simulink model "DCCurrentEstimationslx"  (R2022b)
settings: Solver=ode1  StartTime=0.0  StopTime=0.2  FixedStep=ctrlConst.TsSwitch  MaxStep=1e-6  RelTol=1e-3  EnableMultiTasking=on
undefined symbols (not defined in the file or in its folder): DeadPrd_P, f32_P_Tonoff, f32_P_Tonoff2, Ts
libraries: simulink x5
settings Model: Creator=M00039784  LastModifiedBy=M00039784
settings SolverCC: AlgebraicLoopSolver=TrustRegion  InsertRTBMode=Never (minimum delay)
settings DataIOCC: LimitDataPoints=on  SaveFormat=Array  SaveOutput=off  SaveTime=off
settings OptimizationCC: DefaultParameterBehavior=Inlined  UseDivisionForNetSlopeComputation=on  UseFloatMulNetSlope=on  DefaultUnderspecifiedDataType=single  InlineInvariantSignals=on  PassReuseOutputArgsAs=Individual arguments  ExpressionDepthLimit=2147483647  ZeroExternalMemoryAtStartup=off  ZeroInternalMemoryAtStartup=off  NoFixptDivByZeroProtection=on  EfficientFloat2IntCast=on  LifeSpan=1  EfficientTunableParamExpr=on
settings DebuggingCC: ReadBeforeWriteMsg=DisableAll  WriteAfterWriteMsg=DisableAll  WriteAfterReadMsg=DisableAll  AlgebraicLoopMsg=none  MultiTaskDSMMsg=none  SingleTaskRateTransMsg=error  IntegerOverflowMsg=none  ParameterPrecisionLossMsg=none  FcnCallInpInsideContextMsg=warning  BusObjectLabelMismatch=none  AssertControl=DisableAll  AllowSymbolicDim=off  StateNameClashWarn=warning  SFUnexpectedBacktrackingDiag=warning  SFNoUnconditionalDefaultTransitionDiag=warning  SFExecutionAtInitializationDiag=none  SFMachineParentedDataDiag=warning  IntegerSaturationMsg=none  UnitsInconsistencyMsg=none  ArithmeticOperatorsInVariantConditions=warning
settings HardwareCC: ProdBitPerPointer=32  ProdBitPerSizeT=32  ProdBitPerPtrDiffT=32  ProdLargestAtomicFloat=None  ProdWordSize=32  ProdHWDeviceType=Infineon->TriCore
settings ModelReferenceCC: UpdateModelReferenceTargets=IfOutOfDate  EnableRefExpFcnMdlSchedulingChecks=on  ModelReferenceNumInstancesAllowed=Single  PropagateSignalLabelsOutOfModel=off
settings SFSimCC: SFSimEcho=off  SimUseLocalCustomCode=off  MATLABDynamicMemAlloc=off  CustomCodeUndefinedFunction=UseInterfaceOnly
settings RTWCC: Description=Embedded Coder  SystemTargetFile=ert.tlc  GenCodeOnly=on  GenerateMakefile=off  TemplateMakefile=ec_target.tmf  RTWVerbose=off  RTWUseLocalCustomCode=off  PortableWordSizes=on  CodeExecutionProfiling=on  CodeProfilingSaveOptions=AllData  CodeProfilingInstrumentation=detailed
settings CodeAppCC: ForceParamTrailComments=on  IgnoreCustomStorageClasses=off  IgnoreTestpoints=on  MaxIdLength=64  SimulinkDataObjDesc=on  MATLABFcnDesc=on  CustomSymbolStrGlobalVar=pmsmfoc_rt$N$M  CustomSymbolStrType=pmsmfoc_$N$M  CustomSymbolStrFcn=$N$M$F  CustomSymbolStrFcnArg=$I$N$M  CustomSymbolStrMacro=$N$M  InsertBlockDesc=on  StateflowObjectComments=on  MATLABSourceComments=on  InternalIdentifier=Classic
settings ERTTargetCC: UtilityFuncGeneration=Shared location  MultiwordLength=2048  CombineSignalStateStructs=on  SupportAbsoluteTime=off  SupportNonFinite=off  SupportComplex=off  SupportNonInlinedSFcns=on  RemoveResetFunc=off  ParenthesesLevel=Maximum  GenerateASAP2=on  InlinedParameterPlacement=NonHierarchical  ERTCustomFileTemplate=example_file_process.tlc  EnableDataOwnership=on  ConvertIfToSwitch=off  SuppressUnreachableDefaultCases=off  MemSecPackage=Simulink  MemSecDataConstants=MemConst  MemSecDataParameters=MemConstVolatile
settings ConfigComp: CovMetricSettings=dcmtrzow  CovHTMLOptions=-aTS=1 -bRG=1 -bTC=1 -hTR=0 -nFC=0 -scm=1 -bcm=1 -xEv=0  CovSaveCumulativeToWorkspaceVar=on  CovSaveSingleToWorkspaceVar=on  CovExternalEMLEnable=off  CovSFcnEnable=off
settings SimscapeCC: SimscapeNormalizeSystem=off

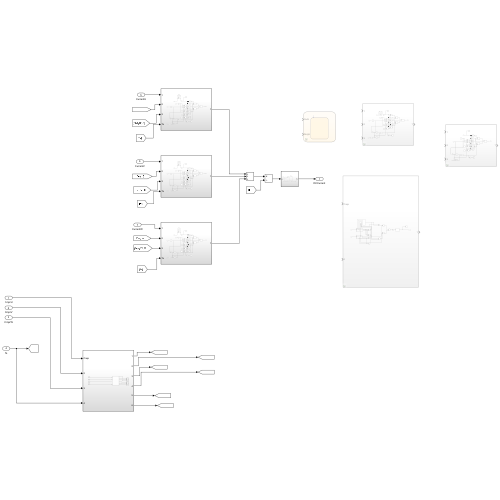
[thumbnail: Simulink's stored preview of the top-level diagram]
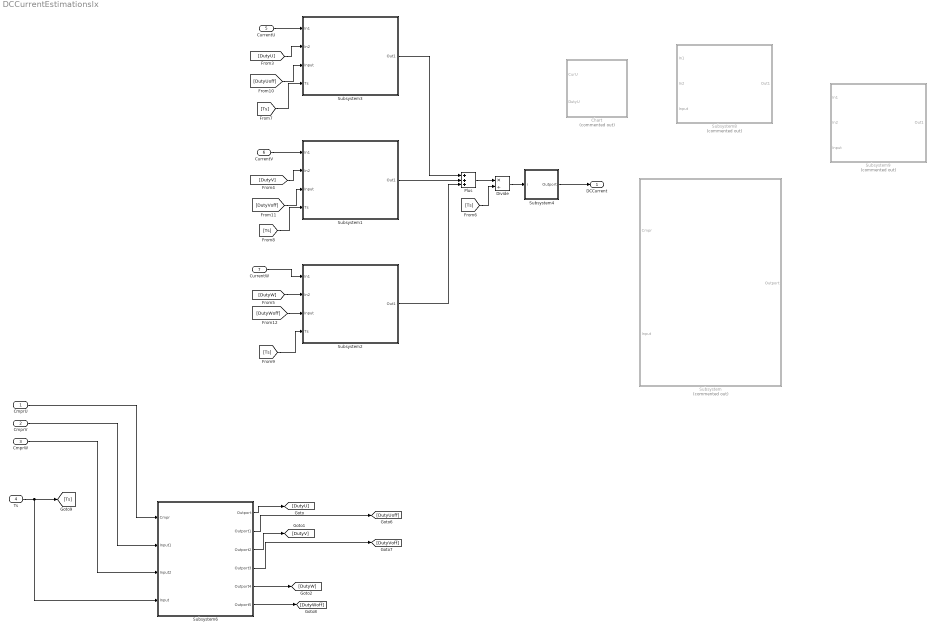
== system DCCurrentEstimationslx ==
  CmprU : Inport  OutDataTypeStr=single  PortDimensions=1  SampleTime=[0.0001,0]
  CmprV : Inport  Port=2  OutDataTypeStr=single
  CmprW : Inport  Port=3  OutDataTypeStr=single
  Ts : Inport  Port=4  OutDataTypeStr=single  PortDimensions=1  SampleTime=[0.0001,0]
  CurrentU : Inport  Port=5  OutDataTypeStr=single
  CurrentV : Inport  Port=6  OutDataTypeStr=single
  CurrentW : Inport  Port=7  OutDataTypeStr=single
  Chart : Stateflow chart  Commented=on  TreatAsAtomicUnit=on
  Divide : Product  Inputs=*/  OutDataTypeStr=single
  Plus : Sum  Inputs=+++
  Subsystem : Subsystem  Commented=on
  Subsystem1 : Subsystem
  Subsystem2 : Subsystem
  Subsystem3 : Subsystem
  Subsystem4 : Subsystem
  Subsystem6 : Subsystem
  Subsystem8 : Subsystem  Commented=on
  Subsystem9 : Subsystem  Commented=on
  DCCurrent : Outport  OutDataTypeStr=single  PortDimensions=1  SampleTime=[0.0001,0]
  wires:
  [DutyU] -> Subsystem3/2(In2)
  CurrentU/1 -> Subsystem3/1(In1)
  CurrentV/1 -> Subsystem1/1(In1)
  [DutyV] -> Subsystem1/2(In2)
  Subsystem1/1(Out1) -> Plus/2
  Plus/1 -> Divide/1
  CurrentW/1 -> Subsystem2/1(In1)
  [DutyW] -> Subsystem2/2(In2)
  Subsystem2/1(Out1) -> Plus/3
  Divide/1 -> Subsystem4/1(i)
  Subsystem4/1(Outport) -> DCCurrent/1
  Subsystem3/1(Out1) -> Plus/1
  [DutyUoff] -> Subsystem3/3(Input)
  [DutyVoff] -> Subsystem1/3(Input)
  [DutyWoff] -> Subsystem2/3(Input)
  Ts/1 -> Subsystem6/4(Input), [Ts]
  [Ts] -> Divide/2
  [Ts] -> Subsystem2/4(Ts)
  [Ts] -> Subsystem3/4(Ts)
  [Ts] -> Subsystem1/4(Ts)
  CmprU/1 -> Subsystem6/1(Cmpr)
  CmprV/1 -> Subsystem6/2(Input1)
  CmprW/1 -> Subsystem6/3(Input2)
  Subsystem6/5(Outport4) -> [DutyW]
  Subsystem6/3(Outport2) -> [DutyV]
  Subsystem6/1(Outport) -> [DutyU]
  Subsystem6/2(Outport1) -> [DutyUoff]
  Subsystem6/4(Outport3) -> [DutyVoff]
  Subsystem6/6(Outport5) -> [DutyWoff]

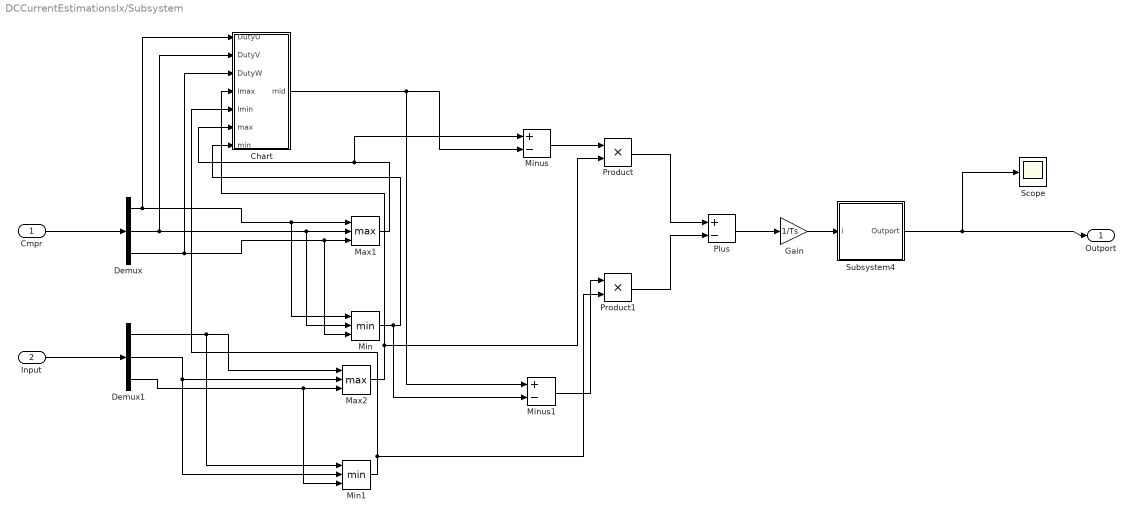
== system DCCurrentEstimationslx/Subsystem ==
  Cmpr : Inport
  Input : Inport  Port=2
  Chart : Stateflow chart  TreatAsAtomicUnit=on
  Demux : Demux  Outputs=3
  Demux1 : Demux  Outputs=3
  Gain : Gain  Gain=1/Ts
  Max1 : MinMax  Function=max  Inputs=3
  Max2 : MinMax  Function=max  Inputs=3
  Min : MinMax  Inputs=3
  Min1 : MinMax  Inputs=3
  Minus : Sum  Inputs=+-
  Minus1 : Sum  Inputs=+-
  Plus : Sum  Inputs=+-
  Product : Product
  Product1 : Product
  Scope : Scope
  Subsystem4 : Subsystem
  Outport : Outport
  wires:
  Subsystem4/1(Outport) -> Outport/1, Scope/1
  Gain/1 -> Subsystem4/1(i)
  Plus/1 -> Gain/1
  Product1/1 -> Plus/2
  Product/1 -> Plus/1
  Minus1/1 -> Product1/1
  Minus/1 -> Product/1
  Chart/1(mid) -> Minus/2, Minus1/1
  Min1/1 -> Chart/5(Imin), Product1/2
  Max2/1 -> Chart/4(Imax), Product/2
  Demux1/1 -> Max2/1, Min1/1
  Demux1/2 -> Max2/2, Min1/2
  Demux1/3 -> Min1/3, Max2/3
  Max1/1 -> Chart/6(max), Minus/1
  Min/1 -> Chart/7(min), Minus1/2
  Demux/1 -> Max1/1, Min/1, Chart/1(DutyU)
  Demux/2 -> Min/2, Max1/2, Chart/2(DutyV)
  Demux/3 -> Max1/3, Min/3, Chart/3(DutyW)
  Input/1 -> Demux1/1
  Cmpr/1 -> Demux/1

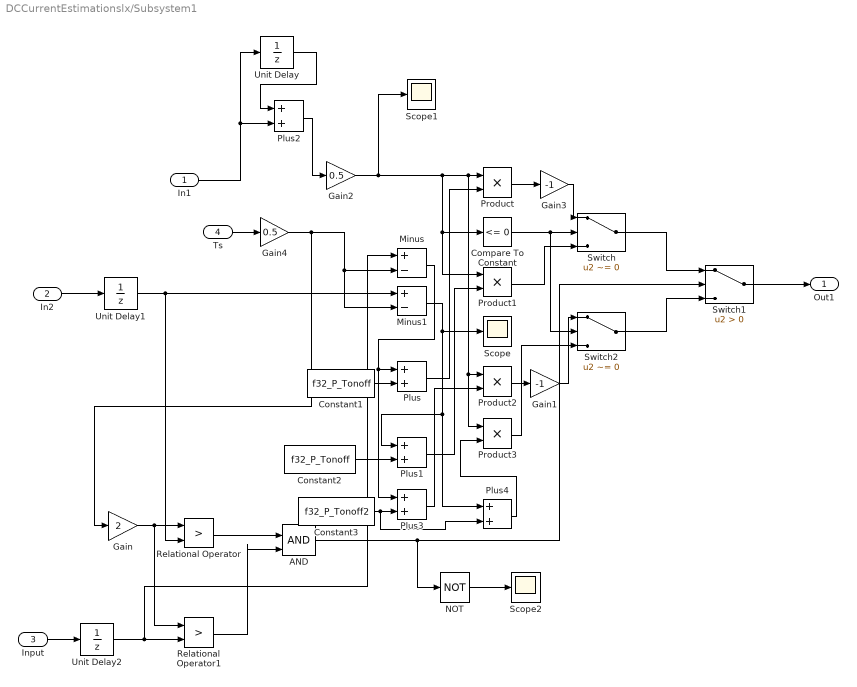
== system DCCurrentEstimationslx/Subsystem1 ==
  In1 : Inport
  In2 : Inport  Port=2
  Input : Inport  Port=3
  Ts : Inport  Port=4
  AND : Logic  IconShape=distinctive  AllPortsSameDT=off  OutDataTypeStr=boolean
  Compare To Constant : simulink/Logic and Bit Operations/Compare To Constant  relop=<=  const=0  OutDataTypeStr=boolean
  Constant1 : Constant  Value=f32_P_Tonoff  OutDataTypeStr=single
  Constant2 : Constant  Value=f32_P_Tonoff  OutDataTypeStr=single
  Constant3 : Constant  Value=f32_P_Tonoff2  OutDataTypeStr=single
  Gain : Gain  Gain=2
  Gain1 : Gain  Gain=-1
  Gain2 : Gain  Gain=0.5
  Gain3 : Gain  Gain=-1
  Gain4 : Gain  Gain=0.5
  Minus : Sum  Inputs=+-
  Minus1 : Sum  Inputs=+-
  NOT : Logic  Operator=NOT  IconShape=distinctive  AllPortsSameDT=off  OutDataTypeStr=boolean
  Plus{,1..4} (5 alike) : Sum
  Product{,1..3} (4 alike) : Product
  Relational Operator : RelationalOperator  Operator=>  OutDataTypeStr=boolean  RndMeth=Simplest  InputSameDT=off
  Relational Operator1 : RelationalOperator  Operator=>  OutDataTypeStr=boolean  RndMeth=Simplest  InputSameDT=off
  Scope : Scope
  Scope1 : Scope
  Scope2 : Scope
  Switch : Switch  Criteria=u2 ~= 0  SaturateOnIntegerOverflow=off  InputSameDT=off
  Switch1 : Switch  Criteria=u2 > Threshold  SaturateOnIntegerOverflow=off  InputSameDT=off
  Switch2 : Switch  Criteria=u2 ~= 0  SaturateOnIntegerOverflow=off  InputSameDT=off
  Unit Delay : UnitDelay  SampleTime=-1  HasFrameUpgradeWarning=on
  Unit Delay1 : UnitDelay  SampleTime=-1  HasFrameUpgradeWarning=on
  Unit Delay2 : UnitDelay  SampleTime=-1  HasFrameUpgradeWarning=on
  Out1 : Outport
  wires:
  Ts/1 -> Gain4/1
  Plus4/1 -> Product3/2
  Plus3/1 -> Product2/2
  Constant3/1 -> Plus3/2, Plus4/2
  Switch2/1 -> Switch1/3
  Plus/1 -> Product/2
  Gain3/1 -> Switch/1
  In1/1 -> Plus2/2, Unit Delay/1
  Unit Delay2/1 -> Relational Operator1/2, Minus/1
  Unit Delay1/1 -> Relational Operator/2, Minus1/1
  Plus2/1 -> Gain2/1
  Unit Delay/1 -> Plus2/1
  NOT/1 -> Scope2/1
  Product3/1 -> Switch2/3
  Gain1/1 -> Switch2/1
  Product2/1 -> Gain1/1
  Switch1/1 -> Out1/1
  Relational Operator1/1 -> AND/2
  Input/1 -> Unit Delay2/1
  Relational Operator/1 -> AND/1
  AND/1 -> Switch1/2, NOT/1
  Gain/1 -> Relational Operator/1, Relational Operator1/1
  Plus1/1 -> Product1/2
  Minus1/1 -> Plus1/1, Plus4/1, Scope/1
  Constant2/1 -> Plus1/2
  Constant1/1 -> Plus/2
  Product1/1 -> Switch/3
  Minus/1 -> Plus3/1, Plus/1
  Compare To Constant/1 -> Switch/2, Switch2/2
  Gain2/1 -> Product/1, Product3/1, Product2/1, Compare To Constant/1, Product1/1, Scope1/1
  Product/1 -> Gain3/1
  Gain4/1 -> Minus1/2, Minus/2, Gain/1
  Switch/1 -> Switch1/1
  In2/1 -> Unit Delay1/1

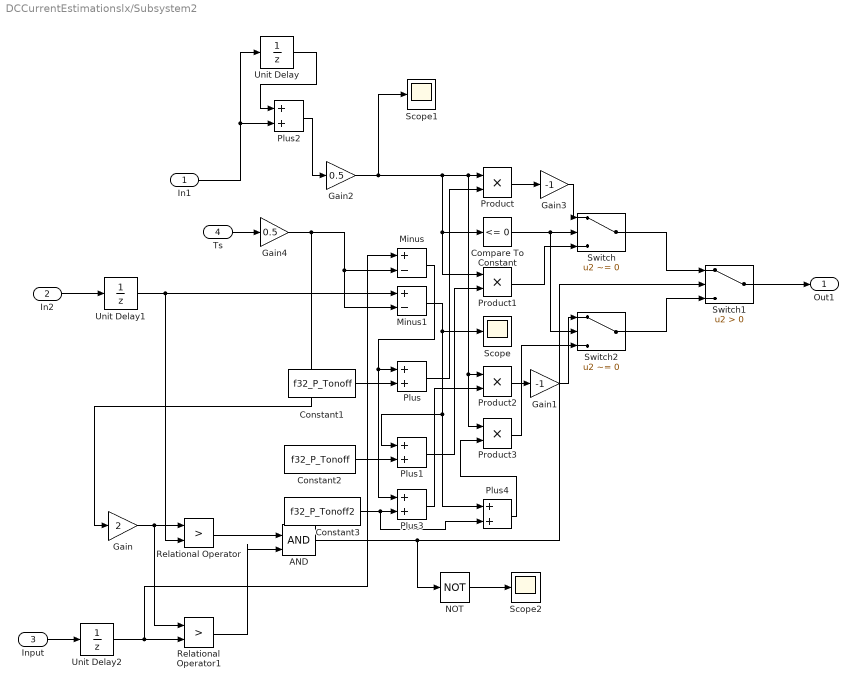
== system DCCurrentEstimationslx/Subsystem2 ==
  In1 : Inport
  In2 : Inport  Port=2
  Input : Inport  Port=3
  Ts : Inport  Port=4
  AND : Logic  IconShape=distinctive  AllPortsSameDT=off  OutDataTypeStr=boolean
  Compare To Constant : simulink/Logic and Bit Operations/Compare To Constant  relop=<=  const=0  OutDataTypeStr=boolean
  Constant1 : Constant  Value=f32_P_Tonoff  OutDataTypeStr=single
  Constant2 : Constant  Value=f32_P_Tonoff  OutDataTypeStr=single
  Constant3 : Constant  Value=f32_P_Tonoff2  OutDataTypeStr=single
  Gain : Gain  Gain=2
  Gain1 : Gain  Gain=-1
  Gain2 : Gain  Gain=0.5
  Gain3 : Gain  Gain=-1
  Gain4 : Gain  Gain=0.5
  Minus : Sum  Inputs=+-
  Minus1 : Sum  Inputs=+-
  NOT : Logic  Operator=NOT  IconShape=distinctive  AllPortsSameDT=off  OutDataTypeStr=boolean
  Plus{,1..4} (5 alike) : Sum
  Product{,1..3} (4 alike) : Product
  Relational Operator : RelationalOperator  Operator=>  OutDataTypeStr=boolean  RndMeth=Simplest  InputSameDT=off
  Relational Operator1 : RelationalOperator  Operator=>  OutDataTypeStr=boolean  RndMeth=Simplest  InputSameDT=off
  Scope : Scope
  Scope1 : Scope
  Scope2 : Scope
  Switch : Switch  Criteria=u2 ~= 0  SaturateOnIntegerOverflow=off  InputSameDT=off
  Switch1 : Switch  Criteria=u2 > Threshold  SaturateOnIntegerOverflow=off  InputSameDT=off
  Switch2 : Switch  Criteria=u2 ~= 0  SaturateOnIntegerOverflow=off  InputSameDT=off
  Unit Delay : UnitDelay  SampleTime=-1  HasFrameUpgradeWarning=on
  Unit Delay1 : UnitDelay  SampleTime=-1  HasFrameUpgradeWarning=on
  Unit Delay2 : UnitDelay  SampleTime=-1  HasFrameUpgradeWarning=on
  Out1 : Outport
  wires:
  Ts/1 -> Gain4/1
  Plus4/1 -> Product3/2
  Plus3/1 -> Product2/2
  Constant3/1 -> Plus3/2, Plus4/2
  Switch2/1 -> Switch1/3
  Plus/1 -> Product/2
  Gain3/1 -> Switch/1
  In1/1 -> Plus2/2, Unit Delay/1
  Unit Delay2/1 -> Relational Operator1/2, Minus/1
  Unit Delay1/1 -> Relational Operator/2, Minus1/1
  Plus2/1 -> Gain2/1
  Unit Delay/1 -> Plus2/1
  NOT/1 -> Scope2/1
  Product3/1 -> Switch2/3
  Gain1/1 -> Switch2/1
  Product2/1 -> Gain1/1
  Switch1/1 -> Out1/1
  Relational Operator1/1 -> AND/2
  Input/1 -> Unit Delay2/1
  Relational Operator/1 -> AND/1
  AND/1 -> Switch1/2, NOT/1
  Gain/1 -> Relational Operator/1, Relational Operator1/1
  Plus1/1 -> Product1/2
  Minus1/1 -> Plus1/1, Plus4/1, Scope/1
  Constant2/1 -> Plus1/2
  Constant1/1 -> Plus/2
  Product1/1 -> Switch/3
  Minus/1 -> Plus3/1, Plus/1
  Compare To Constant/1 -> Switch/2, Switch2/2
  Gain2/1 -> Product/1, Product3/1, Product2/1, Compare To Constant/1, Product1/1, Scope1/1
  Product/1 -> Gain3/1
  Gain4/1 -> Minus1/2, Minus/2, Gain/1
  Switch/1 -> Switch1/1
  In2/1 -> Unit Delay1/1

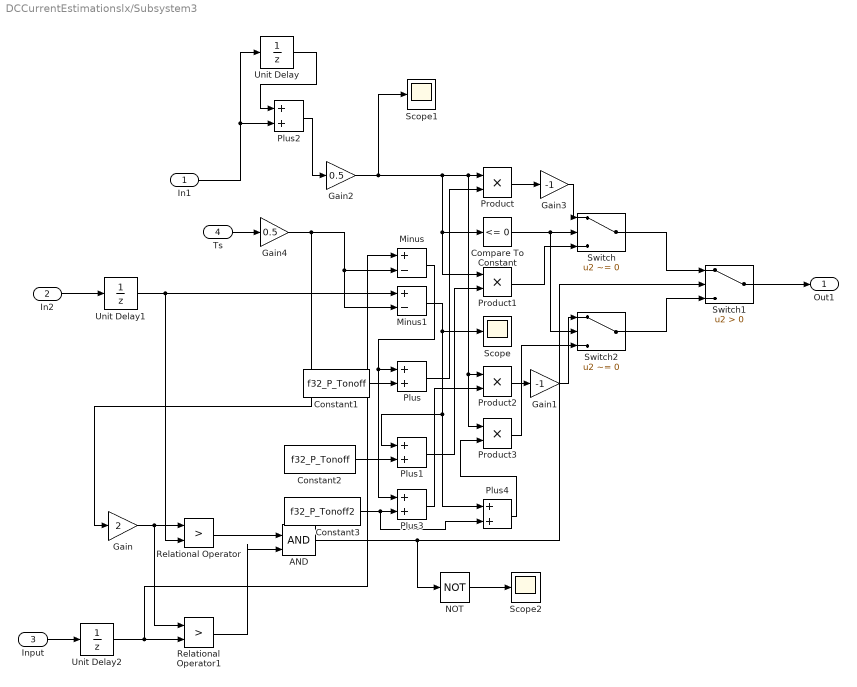
== system DCCurrentEstimationslx/Subsystem3 ==
  In1 : Inport
  In2 : Inport  Port=2
  Input : Inport  Port=3
  Ts : Inport  Port=4
  AND : Logic  IconShape=distinctive  AllPortsSameDT=off  OutDataTypeStr=boolean
  Compare To Constant : simulink/Logic and Bit Operations/Compare To Constant  relop=<=  const=0  OutDataTypeStr=boolean
  Constant1 : Constant  Value=f32_P_Tonoff  OutDataTypeStr=single
  Constant2 : Constant  Value=f32_P_Tonoff  OutDataTypeStr=single
  Constant3 : Constant  Value=f32_P_Tonoff2  OutDataTypeStr=single
  Gain : Gain  Gain=2
  Gain1 : Gain  Gain=-1
  Gain2 : Gain  Gain=0.5
  Gain3 : Gain  Gain=-1
  Gain4 : Gain  Gain=0.5
  Minus : Sum  Inputs=+-
  Minus1 : Sum  Inputs=+-
  NOT : Logic  Operator=NOT  IconShape=distinctive  AllPortsSameDT=off  OutDataTypeStr=boolean
  Plus{,1..4} (5 alike) : Sum
  Product{,1..3} (4 alike) : Product
  Relational Operator : RelationalOperator  Operator=>  OutDataTypeStr=boolean  RndMeth=Simplest  InputSameDT=off
  Relational Operator1 : RelationalOperator  Operator=>  OutDataTypeStr=boolean  RndMeth=Simplest  InputSameDT=off
  Scope : Scope
  Scope1 : Scope
  Scope2 : Scope
  Switch : Switch  Criteria=u2 ~= 0  SaturateOnIntegerOverflow=off  InputSameDT=off
  Switch1 : Switch  Criteria=u2 > Threshold  SaturateOnIntegerOverflow=off  InputSameDT=off
  Switch2 : Switch  Criteria=u2 ~= 0  SaturateOnIntegerOverflow=off  InputSameDT=off
  Unit Delay : UnitDelay  SampleTime=-1  HasFrameUpgradeWarning=on
  Unit Delay1 : UnitDelay  SampleTime=-1  HasFrameUpgradeWarning=on
  Unit Delay2 : UnitDelay  SampleTime=-1  HasFrameUpgradeWarning=on
  Out1 : Outport
  wires:
  Ts/1 -> Gain4/1
  Plus4/1 -> Product3/2
  Plus3/1 -> Product2/2
  Constant3/1 -> Plus3/2, Plus4/2
  Switch2/1 -> Switch1/3
  Plus/1 -> Product/2
  Gain3/1 -> Switch/1
  In1/1 -> Plus2/2, Unit Delay/1
  Unit Delay2/1 -> Relational Operator1/2, Minus/1
  Unit Delay1/1 -> Relational Operator/2, Minus1/1
  Plus2/1 -> Gain2/1
  Unit Delay/1 -> Plus2/1
  NOT/1 -> Scope2/1
  Product3/1 -> Switch2/3
  Gain1/1 -> Switch2/1
  Product2/1 -> Gain1/1
  Switch1/1 -> Out1/1
  Relational Operator1/1 -> AND/2
  Input/1 -> Unit Delay2/1
  Relational Operator/1 -> AND/1
  AND/1 -> Switch1/2, NOT/1
  Gain/1 -> Relational Operator/1, Relational Operator1/1
  Plus1/1 -> Product1/2
  Minus1/1 -> Plus1/1, Plus4/1, Scope/1
  Constant2/1 -> Plus1/2
  Constant1/1 -> Plus/2
  Product1/1 -> Switch/3
  Minus/1 -> Plus3/1, Plus/1
  Compare To Constant/1 -> Switch/2, Switch2/2
  Gain2/1 -> Product/1, Product3/1, Product2/1, Compare To Constant/1, Product1/1, Scope1/1
  Product/1 -> Gain3/1
  Gain4/1 -> Minus1/2, Minus/2, Gain/1
  Switch/1 -> Switch1/1
  In2/1 -> Unit Delay1/1

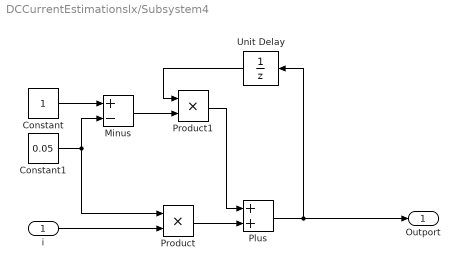
== system DCCurrentEstimationslx/Subsystem4 ==
  i : Inport
  Constant : Constant  OutDataTypeStr=single
  Constant1 : Constant  Value=0.05  OutDataTypeStr=single
  Minus : Sum  Inputs=+-
  Plus : Sum
  Product : Product
  Product1 : Product
  Unit Delay : UnitDelay  SampleTime=-1  HasFrameUpgradeWarning=on
  Outport : Outport
  wires:
  Unit Delay/1 -> Product1/1
  Plus/1 -> Outport/1, Unit Delay/1
  Product1/1 -> Plus/1
  Minus/1 -> Product1/2
  Product/1 -> Plus/2
  i/1 -> Product/2
  Constant1/1 -> Minus/2, Product/1
  Constant/1 -> Minus/1

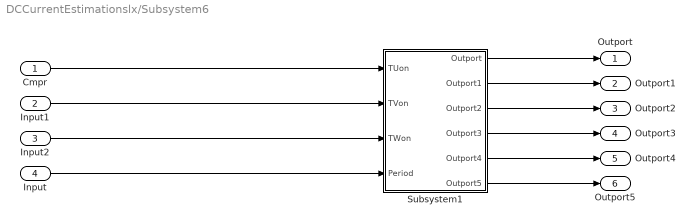
== system DCCurrentEstimationslx/Subsystem6 ==
  Cmpr : Inport
  Input1 : Inport  Port=2
  Input2 : Inport  Port=3
  Input : Inport  Port=4
  Subsystem1 : Subsystem
  Outport : Outport
  Outport1 : Outport  Port=2
  Outport2 : Outport  Port=3
  Outport3 : Outport  Port=4
  Outport4 : Outport  Port=5
  Outport5 : Outport  Port=6
  wires:
  Subsystem1/6(Outport5) -> Outport5/1
  Subsystem1/5(Outport4) -> Outport4/1
  Subsystem1/4(Outport3) -> Outport3/1
  Subsystem1/3(Outport2) -> Outport2/1
  Subsystem1/2(Outport1) -> Outport1/1
  Subsystem1/1(Outport) -> Outport/1
  Input/1 -> Subsystem1/4(Period)
  Input2/1 -> Subsystem1/3(TWon)
  Input1/1 -> Subsystem1/2(TVon)
  Cmpr/1 -> Subsystem1/1(TUon)

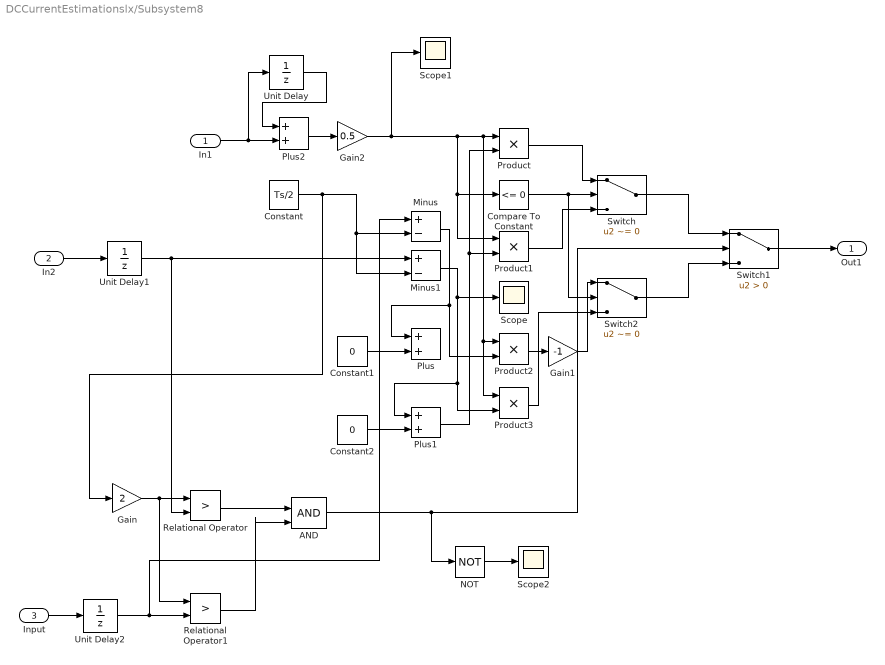
== system DCCurrentEstimationslx/Subsystem8 ==
  In1 : Inport
  In2 : Inport  Port=2
  Input : Inport  Port=3
  AND : Logic  IconShape=distinctive  AllPortsSameDT=off  OutDataTypeStr=boolean
  Compare To Constant : simulink/Logic and Bit Operations/Compare To Constant  relop=<=  const=0  OutDataTypeStr=boolean
  Constant : Constant  Value=Ts/2
  Constant1 : Constant  Value=0
  Constant2 : Constant  Value=0
  Gain : Gain  Gain=2
  Gain1 : Gain  Gain=-1
  Gain2 : Gain  Gain=0.5
  Minus : Sum  Inputs=+-
  Minus1 : Sum  Inputs=+-
  NOT : Logic  Operator=NOT  IconShape=distinctive  AllPortsSameDT=off  OutDataTypeStr=boolean
  Plus : Sum
  Plus1 : Sum
  Plus2 : Sum
  Product{,1..3} (4 alike) : Product
  Relational Operator : RelationalOperator  Operator=>  OutDataTypeStr=boolean  RndMeth=Simplest  InputSameDT=off
  Relational Operator1 : RelationalOperator  Operator=>  OutDataTypeStr=boolean  RndMeth=Simplest  InputSameDT=off
  Scope : Scope
  Scope1 : Scope
  Scope2 : Scope
  Switch : Switch  Criteria=u2 ~= 0  SaturateOnIntegerOverflow=off  InputSameDT=off
  Switch1 : Switch  Criteria=u2 > Threshold  SaturateOnIntegerOverflow=off  InputSameDT=off
  Switch2 : Switch  Criteria=u2 ~= 0  SaturateOnIntegerOverflow=off  InputSameDT=off
  Unit Delay : UnitDelay  SampleTime=-1  HasFrameUpgradeWarning=on
  Unit Delay1 : UnitDelay  SampleTime=-1  HasFrameUpgradeWarning=on
  Unit Delay2 : UnitDelay  SampleTime=-1  HasFrameUpgradeWarning=on
  Out1 : Outport
  wires:
  In1/1 -> Plus2/2, Unit Delay/1
  Unit Delay2/1 -> Relational Operator1/2, Minus/1
  Unit Delay1/1 -> Relational Operator/2, Minus1/1
  Plus2/1 -> Gain2/1
  Unit Delay/1 -> Plus2/1
  NOT/1 -> Scope2/1
  Product3/1 -> Switch2/3
  Gain1/1 -> Switch2/1
  Product2/1 -> Gain1/1
  Switch1/1 -> Out1/1
  Switch2/1 -> Switch1/3
  Relational Operator1/1 -> AND/2
  Input/1 -> Unit Delay2/1
  Relational Operator/1 -> AND/1
  AND/1 -> Switch1/2, NOT/1
  Gain/1 -> Relational Operator/1, Relational Operator1/1
  Plus1/1 -> Product/2, Product1/2
  Minus1/1 -> Plus1/1, Product3/2, Scope/1
  Constant2/1 -> Plus1/2
  Constant1/1 -> Plus/2
  Product1/1 -> Switch/3
  Minus/1 -> Plus/1, Product2/2
  Compare To Constant/1 -> Switch/2, Switch2/2
  Gain2/1 -> Product/1, Product3/1, Product2/1, Compare To Constant/1, Product1/1, Scope1/1
  Product/1 -> Switch/1
  Constant/1 -> Minus1/2, Minus/2, Gain/1
  Switch/1 -> Switch1/1
  In2/1 -> Unit Delay1/1

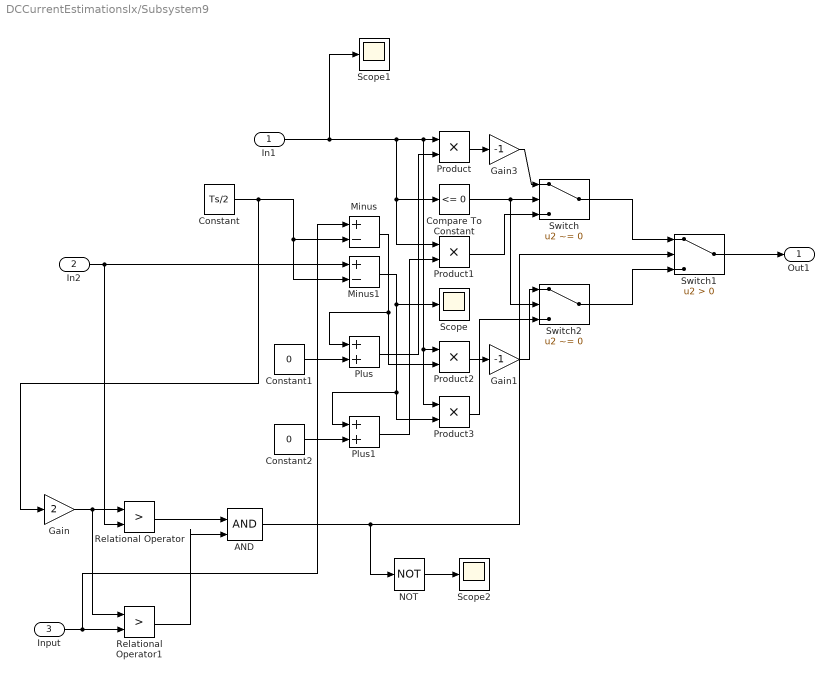
== system DCCurrentEstimationslx/Subsystem9 ==
  In1 : Inport
  In2 : Inport  Port=2
  Input : Inport  Port=3
  AND : Logic  IconShape=distinctive  AllPortsSameDT=off  OutDataTypeStr=boolean
  Compare To Constant : simulink/Logic and Bit Operations/Compare To Constant  relop=<=  const=0  OutDataTypeStr=boolean
  Constant : Constant  Value=Ts/2
  Constant1 : Constant  Value=0
  Constant2 : Constant  Value=0
  Gain : Gain  Gain=2
  Gain1 : Gain  Gain=-1
  Gain3 : Gain  Gain=-1
  Minus : Sum  Inputs=+-
  Minus1 : Sum  Inputs=+-
  NOT : Logic  Operator=NOT  IconShape=distinctive  AllPortsSameDT=off  OutDataTypeStr=boolean
  Plus : Sum
  Plus1 : Sum
  Product{,1..3} (4 alike) : Product
  Relational Operator : RelationalOperator  Operator=>  OutDataTypeStr=boolean  RndMeth=Simplest  InputSameDT=off
  Relational Operator1 : RelationalOperator  Operator=>  OutDataTypeStr=boolean  RndMeth=Simplest  InputSameDT=off
  Scope : Scope
  Scope1 : Scope
  Scope2 : Scope
  Switch : Switch  Criteria=u2 ~= 0  SaturateOnIntegerOverflow=off  InputSameDT=off
  Switch1 : Switch  Criteria=u2 > Threshold  SaturateOnIntegerOverflow=off  InputSameDT=off
  Switch2 : Switch  Criteria=u2 ~= 0  SaturateOnIntegerOverflow=off  InputSameDT=off
  Out1 : Outport
  wires:
  NOT/1 -> Scope2/1
  Product3/1 -> Switch2/3
  Gain1/1 -> Switch2/1
  Product2/1 -> Gain1/1
  Switch1/1 -> Out1/1
  Switch2/1 -> Switch1/3
  Relational Operator1/1 -> AND/2
  Input/1 -> Relational Operator1/2, Minus/1
  Relational Operator/1 -> AND/1
  AND/1 -> Switch1/2, NOT/1
  Gain/1 -> Relational Operator/1, Relational Operator1/1
  Plus1/1 -> Product1/2
  Minus1/1 -> Plus1/1, Product3/2, Scope/1
  Constant2/1 -> Plus1/2
  Plus/1 -> Product/2
  Constant1/1 -> Plus/2
  Product1/1 -> Switch/3
  Product/1 -> Gain3/1
  Minus/1 -> Plus/1, Product2/2
  Compare To Constant/1 -> Switch/2, Switch2/2
  In1/1 -> Product/1, Product3/1, Product2/1, Compare To Constant/1, Product1/1, Scope1/1
  Gain3/1 -> Switch/1
  Constant/1 -> Minus1/2, Minus/2, Gain/1
  Switch/1 -> Switch1/1
  In2/1 -> Relational Operator/2, Minus1/1

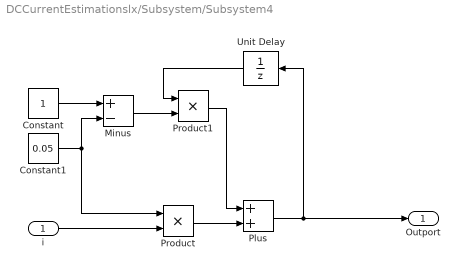
== system DCCurrentEstimationslx/Subsystem/Subsystem4 ==
  i : Inport
  Constant : Constant
  Constant1 : Constant  Value=0.05
  Minus : Sum  Inputs=+-
  Plus : Sum
  Product : Product
  Product1 : Product
  Unit Delay : UnitDelay  SampleTime=-1  HasFrameUpgradeWarning=on
  Outport : Outport
  wires:
  Unit Delay/1 -> Product1/1
  Plus/1 -> Outport/1, Unit Delay/1
  Product1/1 -> Plus/1
  Minus/1 -> Product1/2
  Product/1 -> Plus/2
  i/1 -> Product/2
  Constant1/1 -> Minus/2, Product/1
  Constant/1 -> Minus/1

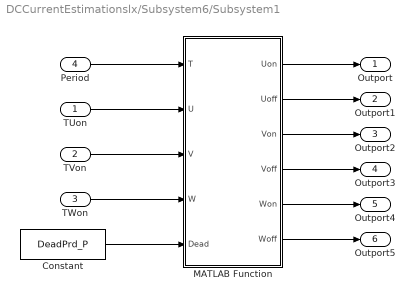
== system DCCurrentEstimationslx/Subsystem6/Subsystem1 ==
  TUon : Inport
  TVon : Inport  Port=2
  TWon : Inport  Port=3
  Period : Inport  Port=4
  Constant : Constant  Value=DeadPrd_P  OutDataTypeStr=single
  MATLAB Function : MATLAB Function  TreatAsAtomicUnit=on
  Outport : Outport  OutDataTypeStr=single
  Outport1 : Outport  Port=2  OutDataTypeStr=single
  Outport2 : Outport  Port=3  OutDataTypeStr=single
  Outport3 : Outport  Port=4  OutDataTypeStr=single
  Outport4 : Outport  Port=5  OutDataTypeStr=single
  Outport5 : Outport  Port=6  OutDataTypeStr=single
  wires:
  MATLAB Function/6(Woff) -> Outport5/1
  MATLAB Function/5(Won) -> Outport4/1
  MATLAB Function/4(Voff) -> Outport3/1
  MATLAB Function/3(Von) -> Outport2/1
  MATLAB Function/2(Uoff) -> Outport1/1
  MATLAB Function/1(Uon) -> Outport/1
  TWon/1 -> MATLAB Function/4(W)
  TVon/1 -> MATLAB Function/3(V)
  TUon/1 -> MATLAB Function/2(U)
  Period/1 -> MATLAB Function/1(T)
  Constant/1 -> MATLAB Function/5(Dead)

== matlab function DCCurrentEstimationslx/Subsystem6/Subsystem1/MATLAB Function ==
  data: T input; Uon output; U input; V input; W input; Dead input; Uoff output; Von output; Voff output; Won output; Woff output
function [Uon,Uoff,Von,Voff,Won,Woff] = fcn(T,U,V,W,Dead)

TempU = U;%min(U,T);
TempV = V;%min(V,T);
TempW = W;%min(W,T);
Tempmax = T - Dead;
Tempmin = Dead;
if(TempU>Tempmax)
    Uon = T;
    Uoff = single(0);
elseif(TempU<Tempmin)
    Uon = single(0);
    Uoff = T - TempU;
else
    Uon = TempU;
    Uoff = T - TempU;
end

if(TempV>Tempmax)
    Von = T;
    Voff = single(0);
elseif(TempV<Tempmin)
    Von = single(0);
    Voff = T - TempV;
else
    Von = TempV;
    Voff = T - TempV;
end

if(TempW>Tempmax)
    Won = T;
    Woff = single(0);
elseif(TempW<Tempmin)
    Won = single(0);
    Woff = T - TempW;
else
    Won = TempW;
    Woff = T - TempW;
end

== stateflow chart DCCurrentEstimationslx/Chart ==
  state CurUEst
    du:
    if(CurU>=0)
  (default) -> CurUEst
  data: CurU input; DutyU input; Ts local =1e-4

== stateflow chart DCCurrentEstimationslx/Subsystem/Chart ==
  state Init
    en:
    Tempmax=0;
    mid=0;
    Tempmin=0;
    du:
    if(max>DutyU>min)
    mid=DutyU;
    end
    if(max>DutyV>min)
    mid=DutyV;
    end
    if(max>DutyW>min)
    mid=DutyW;
    end
  (default) -> Init
  data: DutyU input; Tempmax local; DutyV input; DutyW input; Imax input; Imin input; Tempmin local; max input; min input; mid output
